simulink model "Hall_sensor_120deg_filter_org"  (R2024b)
settings: Solver=FixedStepAuto  StartTime=0.0  StopTime=1.5  FixedStep=1e-6  RelTol=1e-3
undefined symbols (not defined in the file): closed_loop, control_mode, D_duty_cycle, D_m, DiscIntNeverNeededParam, hall_errors, hall_errors_ON, I_duty_cycle, J_t, L_ss, lambda_m, P, P_duty_cycle, r_s, R_vs, T_m, theta_v, V_bus
libraries: spsMosfetLib x6, spsSeriesRLCBranchLib x4, spsVoltageMeasurementLib x3, spsControlledCurrentSourceLib x3, eeGeneralControl x2, slpidlib x2, embmathops x2, simulink x1, spsPWMGeneratorDCDCLib x1, spsDCVoltageSourceLib x1, sps_lib x1
settings Model: SimulationMode=accelerator  Creator=baolo  LastModifiedBy=baolo
settings SolverCC: ZeroCrossAlgorithm=Adaptive
settings DebuggingCC: IgnoredZcDiagnostic=none

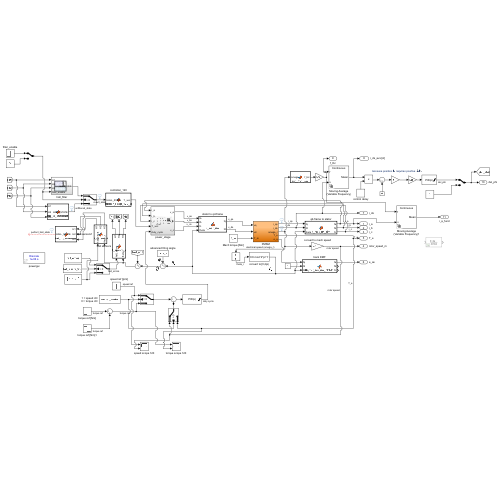
[thumbnail: Simulink's stored preview of the top-level diagram]
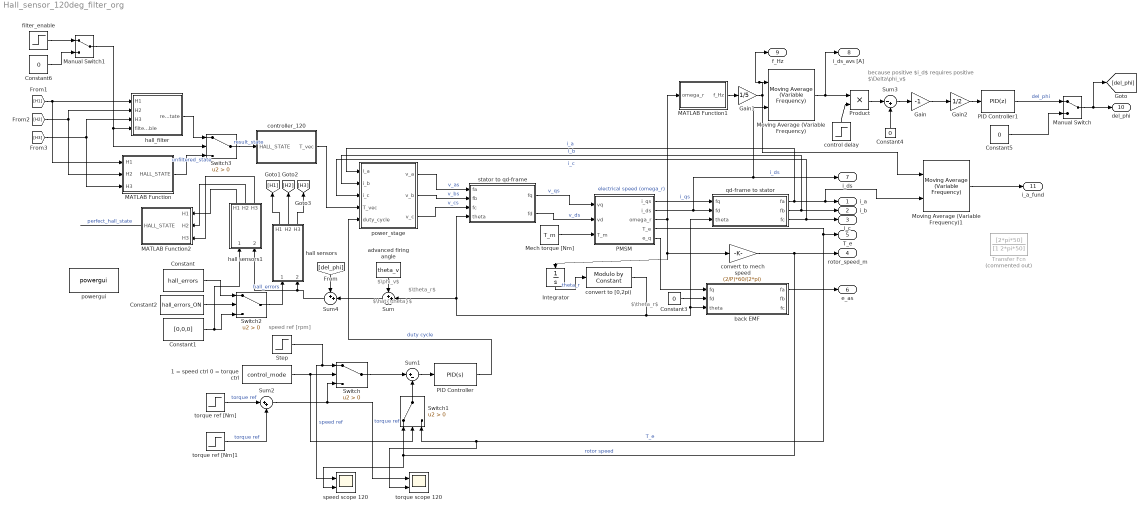
== system Hall_sensor_120deg_filter_org ==
  note: because positive $i_d$ requires positive $\Delta\phi_v$
  note: $\phi_v$
  note: speed ref [rpm]
  note: $\theta_r$
  note: $\theta_r$
  note: $\hat{\theta}$
  1 = speed ctrl 0 = torque ctrl : Constant  Value=control_mode
  Constant : Constant  Value=hall_errors
  Constant1 : Constant  Value=[0,0,0]
  Constant2 : Constant  Value=hall_errors_ON
  Constant{3..6} (4 alike) : Constant  Value=0
  Gain : Gain  Gain=-1
  Gain1 : Gain  Gain=1/5
  Gain2 : Gain  Gain=1/2
  Integrator : Integrator
  MATLAB Function : MATLAB Function  TreatAsAtomicUnit=on
  MATLAB Function1 : MATLAB Function  TreatAsAtomicUnit=on
  MATLAB Function2 : MATLAB Function  TreatAsAtomicUnit=on
  Manual Switch : ManualSwitch
  Manual Switch1 : ManualSwitch
  Mech torque [Nm] : Constant  Value=T_m
  Moving Average (Variable Frequency) : eeGeneralControl/Moving Average (Variable Frequency)  VariantControl=Variant1  LabelModeActiveChoice=Continuous  f0=60  fmin=0.1  x0=0  BufferSize=32768  Ts=0
      settings: LibrarySourceBlock=|
      | ee_sl_lib/General Control/Moving Average
      | (Variable Frequency)
  Moving Average (Variable Frequency)1 : eeGeneralControl/Moving Average (Variable Frequency)  VariantControl=Variant1  LabelModeActiveChoice=Continuous  f0=60  fmin=0.1  x0=0  BufferSize=32768  Ts=0
      settings: LibrarySourceBlock=|
      | ee_sl_lib/General Control/Moving Average
      | (Variable Frequency)
  PID Controller : slpidlib/PID Controller  Controller=PID  Form=Parallel  TimeDomain=Continuous-time  UseExternalTs=off  SampleTime=-1  IntegratorMethod=Forward Euler  FilterMethod=Forward Euler  ControllerParametersSource=internal  P=P_duty_cycle  I=I_duty_cycle  UseKiTs=off  D=D_duty_cycle  UseExternalDerivativeSource=off  N=100  UseFilter=on  TunerSelectOption=Transfer Function Based (PID Tuner App)  InitialConditionSource=internal  InitialConditionForIntegrator=0  InitialConditionForFilter=0  DifferentiatorICPrevScaledInput=0  ExternalReset=none  TrackingMode=off  Kt=1  LimitOutput=on  SatLimitsSource=internal  UpperSaturationLimit=1  LowerSaturationLimit=0  LinearizeAsGain=on  AntiWindupMode=none  Kb=1  LimitIntegrator=off  UpperIntegratorSaturationLimit=inf  LowerIntegratorSaturationLimit=-inf  POutMin=[]  POutMax=[]  IOutMin=[]  IOutMax=[]  DOutMin=[]  DOutMax=[]  NOutMin=[]  NOutMax=[]  SumOutMin=[]  SumOutMax=[]  SaturationOutMin=[]  SaturationOutMax=[]  PParamMin=[]  PParamMax=[]  IParamMin=[]  IParamMax=[]  DParamMin=[]  DParamMax=[]  NParamMin=[]  NParamMax=[]  KbParamMin=[]  KbParamMax=[]  KtParamMin=[]  KtParamMax=[]  KbOutMin=[]  KbOutMax=[]  KtOutMin=[]  KtOutMax=[]  IntegratorOutMin=[]  IntegratorOutMax=[]  FilterOutMin=[]  FilterOutMax=[]  SumI1OutMin=[]  SumI1OutMax=[]  SumI2OutMin=[]  SumI2OutMax=[]  SumI3OutMin=[]  SumI3OutMax=[]  SumI4OutMin=[]  SumI4OutMax=[]  SumDOutMin=[]  SumDOutMax=[]  DifferentiatorOutMin=[]  DifferentiatorOutMax=[]  FilterDiffOutCoefMin=[]  FilterDiffOutCoefMax=[]  ReciprocalOutMin=[]  ReciprocalOutMax=[]  SumDenOutMin=[]  SumDenOutMax=[]  SumNumOutMin=[]  SumNumOutMax=[]  DivideOutMin=[]  DivideOutMax=[]  UdiffTsProdOutMin=[]  UdiffTsProdOutMax=[]  NTsProdOutMin=[]  NTsProdOutMax=[]  UintegralTsProdOutMin=[]  UintegralTsProdOutMax=[]  UngainTsProdOutMin=[]  UngainTsProdOutMax=[]  ClampingZeroOutDataTypeStr=Inherit: Inherit via back propagation  ClampingZeroOutMin=[]  ClampingZeroOutMax=[]  FilterDenConstantOutDataTypeStr=Inherit: Inherit via back propagation  FilterDenConstantOutMin=[]  FilterDenConstantOutMax=[]  PCopyOutDataTypeStr=Inherit: Inherit via back propagation  PCopyOutMin=[]  PCopyOutMax=[]  NCopyOutDataTypeStr=Inherit: Inherit via back propagation  NCopyOutMin=[]  NCopyOutMax=[]  IntegratorContinuousStateAttributes=''  IntegratorStateMustResolveToSignalObject=off  IntegratorRTWStateStorageClass=Auto  FilterContinuousStateAttributes=''  FilterStateMustResolveToSignalObject=off  FilterRTWStateStorageClass=Auto  ParallelPVariant=InternalParameters  IdealPVariant=Disabled  IVariant=InternalParameters  DVariant=InternalParameters  IntegratorVariant=Continuous  SatVariant=Enabled  AWVariant=Passthrough  PCopyVariant=Disabled  TRVariant=Disabled  FdbkBlocksVariant=Forward  IdealPFdbkVariant=Disabled  SatFdbkVariant=Disabled  DerivativeFilterVariant=ContFilter  NVariant=InternalParameters  NCopyVariant=Disabled  FilterICVariant=InternalICsFilter  IntegratorICVariant=InternalICs  ExternalResetVariant=Disabled  TRSumVariant=Passthrough  SumFdbkVariant=Disabled  SumVariant=Sum_PID  TsampFilterVariant=InternalTs  TsampNgainVariant=Passthrough  TsampIntegralVariant=Disabled_SignalSpec  ExternalSaturationOutDataTypeStr=Inherit: Same as second input  DerivativeSourceVariant=ErrorSignal  PreIntVariant=InternalPreInt
  PID Controller1 : slpidlib/PID Controller  Controller=PID  Form=Parallel  TimeDomain=Discrete-time  UseExternalTs=off  SampleTime=-1  IntegratorMethod=Forward Euler  FilterMethod=Forward Euler  ControllerParametersSource=internal  P=0.0136  I=1.488  UseKiTs=off  D=0  UseExternalDerivativeSource=off  N=100  UseFilter=on  TunerSelectOption=Transfer Function Based (PID Tuner App)  InitialConditionSource=internal  InitialConditionForIntegrator=0  InitialConditionForFilter=0  DifferentiatorICPrevScaledInput=0  ExternalReset=none  TrackingMode=off  Kt=1  LimitOutput=on  SatLimitsSource=internal  UpperSaturationLimit=pi/3  LowerSaturationLimit=-pi/3  LinearizeAsGain=on  AntiWindupMode=none  Kb=1  LimitIntegrator=off  UpperIntegratorSaturationLimit=inf  LowerIntegratorSaturationLimit=-inf  POutMin=[]  POutMax=[]  IOutMin=[]  IOutMax=[]  DOutMin=[]  DOutMax=[]  NOutMin=[]  NOutMax=[]  SumOutMin=[]  SumOutMax=[]  SaturationOutMin=[]  SaturationOutMax=[]  PParamMin=[]  PParamMax=[]  IParamMin=[]  IParamMax=[]  DParamMin=[]  DParamMax=[]  NParamMin=[]  NParamMax=[]  KbParamMin=[]  KbParamMax=[]  KtParamMin=[]  KtParamMax=[]  KbOutMin=[]  KbOutMax=[]  KtOutMin=[]  KtOutMax=[]  IntegratorOutMin=[]  IntegratorOutMax=[]  FilterOutMin=[]  FilterOutMax=[]  SumI1OutMin=[]  SumI1OutMax=[]  SumI2OutMin=[]  SumI2OutMax=[]  SumI3OutMin=[]  SumI3OutMax=[]  SumI4OutMin=[]  SumI4OutMax=[]  SumDOutMin=[]  SumDOutMax=[]  DifferentiatorOutMin=[]  DifferentiatorOutMax=[]  FilterDiffOutCoefMin=[]  FilterDiffOutCoefMax=[]  ReciprocalOutMin=[]  ReciprocalOutMax=[]  SumDenOutMin=[]  SumDenOutMax=[]  SumNumOutMin=[]  SumNumOutMax=[]  DivideOutMin=[]  DivideOutMax=[]  UdiffTsProdOutMin=[]  UdiffTsProdOutMax=[]  NTsProdOutMin=[]  NTsProdOutMax=[]  UintegralTsProdOutMin=[]  UintegralTsProdOutMax=[]  UngainTsProdOutMin=[]  UngainTsProdOutMax=[]  ClampingZeroOutDataTypeStr=Inherit: Inherit via back propagation  ClampingZeroOutMin=[]  ClampingZeroOutMax=[]  FilterDenConstantOutDataTypeStr=Inherit: Inherit via back propagation  FilterDenConstantOutMin=[]  FilterDenConstantOutMax=[]  PCopyOutDataTypeStr=Inherit: Inherit via back propagation  PCopyOutMin=[]  PCopyOutMax=[]  NCopyOutDataTypeStr=Inherit: Inherit via back propagation  NCopyOutMin=[]  NCopyOutMax=[]  IntegratorContinuousStateAttributes=''  IntegratorStateMustResolveToSignalObject=off  IntegratorRTWStateStorageClass=Auto  FilterContinuousStateAttributes=''  FilterStateMustResolveToSignalObject=off  FilterRTWStateStorageClass=Auto  ParallelPVariant=InternalParameters  IdealPVariant=Disabled  IVariant=InternalParameters  DVariant=InternalParameters  IntegratorVariant=Discrete  SatVariant=Enabled  AWVariant=Passthrough  PCopyVariant=Disabled  TRVariant=Disabled  FdbkBlocksVariant=Forward  IdealPFdbkVariant=Disabled  SatFdbkVariant=Disabled  DerivativeFilterVariant=ForwardEulerFilter  NVariant=InternalParameters  NCopyVariant=Disabled  FilterICVariant=InternalICsFilter  IntegratorICVariant=InternalICs  ExternalResetVariant=Disabled  TRSumVariant=Passthrough  SumFdbkVariant=Disabled  SumVariant=Sum_PID  TsampFilterVariant=InternalTs  TsampNgainVariant=Passthrough  TsampIntegralVariant=Disabled_SignalSpec  ExternalSaturationOutDataTypeStr=Inherit: Same as second input  DerivativeSourceVariant=ErrorSignal  PreIntVariant=InternalPreInt
  PMSM : Subsystem
  Product : Product
  Step : Step  Time=0.1  After=1000  SampleTime=0
  Sum : Sum  Inputs=++|
  Sum1 : Sum  Inputs=|+-
  Sum2 : Sum  Inputs=|++
  Sum3 : Sum  Inputs=|-+
  Sum4 : Sum  Inputs=++|
  Switch{,1..3} (4 alike) : Switch  Criteria=u2 > Threshold  SaturateOnIntegerOverflow=off  InputSameDT=off
  Transfer Fcn : TransferFcn  Commented=on  Numerator=[2*pi*50]  Denominator=[1 2*pi*50]
  advanced firing angle : Constant  Value=theta_v
  back EMF : MATLAB Function  TreatAsAtomicUnit=on
  control delay : Step  Time=0.7  SampleTime=0
  controller_120 : MATLAB Function  TreatAsAtomicUnit=on
  convert to [0,2pi) : embmathops/Modulo by Constant  Denominator=2*pi  SimulateUsing=Code generation
      settings: LibrarySourceBlock=embeddedMathLib/Modulo by Constant
  convert to mech speed : Gain  Gain=(2/P)*60/(2*pi)
  filter_enable : Step  Time=0.5  SampleTime=0
  hall sensors : MATLAB Function  TreatAsAtomicUnit=on
  hall sensors1 : MATLAB Function  TreatAsAtomicUnit=on
  hall_filter : Subsystem
  power_stage : Subsystem
  powergui : sps_lib/powergui  Priority=1  SimulationMode=Discrete  SampleTime=1e-6  frequency=60  Iterations=50  frequencyindice=0  Pbase=100e6  ErrMax=1e-4  UnitsV=kV  UnitsW=MW  buscounter=0  FunctionMessages=off  echomessages=off  EnableUseOfTLC=off  CurrentSourceSwitches=off  DisableSnubberDevices=off  DisableRonSwitches=off  DisableVfSwitches=off  DisplayEquations=off  AutomaticDiscreteSolvers=off  SolverType=Tustin/Backward Euler (TBE)  Interpol=off  ExternalGateDelay=off  methode=off  Ts=100  x0status=blocks  SPID=on  SwTol=0  HookPort=off  NonlinearTolerance=1e-4  nMaxIteration=100  ContinueOnMaxIteration=off  RestoreLinks=warning  ResistiveCurrentMeasurement=off  Frange=[0:2:500]  Ylog=off  Xlog=on  ShowGrid=off  save=off  variable=ZData  structure=0  ZoomFFT=off  StartTime=0.0  cycles=1  DisplayStyle=1  fundamental=60  FreqAxis=off  MaxFrequency=1000  frequencyindicesteady=1  RmsSteady=1  display=off
  qd-frame to stator : MATLAB Function  TreatAsAtomicUnit=on
  speed scope 120 : Scope  NumInputPorts=2
  stator to qd-frame : MATLAB Function  TreatAsAtomicUnit=on
  torque ref [Nm] : Step  Time=0.1  After=1e-1  SampleTime=0  ZeroCross=off
  torque ref [Nm]1 : Step  After=-0.5e-1  SampleTime=0
  torque scope 120 : Scope  NumInputPorts=2
  i_a : Outport
  i_b : Outport  Port=2
  i_c : Outport  Port=3
  rotor_speed_m : Outport  Port=4
  T_e : Outport  Port=5
  e_as : Outport  Port=6
  i_ds : Outport  Port=7
  i_ds_avs [A] : Outport  Port=8
  f_Hz : Outport  Port=9
  del_phi : Outport  Port=10
  i_a_fund : Outport  Port=11
  wires:
  stator to qd-frame/1(fq) -> PMSM/1(vq)  "v_qs"
  stator to qd-frame/2(fd) -> PMSM/2(vd)  "v_ds"
  Mech torque [Nm]/1 -> PMSM/3(T_m)
  PMSM/1(i_qs) -> qd-frame to stator/1(fq)  "i_qs"
  PMSM/2(i_ds) -> i_ds/1, Moving Average (Variable Frequency)/2, qd-frame to stator/2(fd)  "i_ds"
  PMSM/3(omega_r) -> MATLAB Function1/1(omega_r), convert to mech speed/1, Integrator/1  "electrical speed (omega_r)"
  convert to [0,2pi)/1 -> stator to qd-frame/4(theta), Sum/2, back EMF/3(theta), qd-frame to stator/3(theta)
  power_stage/1(v_a) -> stator to qd-frame/1(fa)  "v_as"
  power_stage/2(v_b) -> stator to qd-frame/2(fb)  "v_bs"
  power_stage/3(v_c) -> stator to qd-frame/3(fc)  "v_cs"
  Integrator/1 -> convert to [0,2pi)/1  "theta_r"
  hall sensors/1(H1) -> [H1]
  hall sensors/2(H2) -> [H2]
  hall sensors/3(H3) -> [H3]
  advanced firing angle/1 -> Sum/1
  Sum/1 -> Sum4/2
  qd-frame to stator/1(fa) -> power_stage/1(i_a), Moving Average (Variable Frequency)1/2, i_a/1  "i_a"
  qd-frame to stator/2(fb) -> power_stage/2(i_b), i_b/1  "i_b"
  qd-frame to stator/3(fc) -> power_stage/3(i_c), i_c/1  "i_c"
  convert to mech speed/1 -> rotor_speed_m/1, speed scope 120/2, Switch1/1  "rotor speed"
  PMSM/4(T_e) -> torque scope 120/2, Switch1/3, T_e/1  "T_e"
  1 = speed ctrl 0 = torque ctrl/1 -> Switch/2, Switch1/2
  Step/1 -> speed scope 120/1, Switch/1  "speed ref"
  Sum2/1 -> torque scope 120/1, Switch/3  "torque ref"
  Switch1/1 -> Sum1/2
  Switch/1 -> Sum1/1
  Sum1/1 -> PID Controller/1
  PID Controller/1 -> power_stage/5(duty_cycle)  "duty cycle"
  torque ref [Nm]/1 -> Sum2/1  "torque ref"
  torque ref [Nm]1/1 -> Sum2/2  "torque ref"
  Constant/1 -> Switch2/1
  Switch2/1 -> hall sensors/1(hall_errors)  "hall_errors"
  Constant1/1 -> hall sensors1/1(hall_errors), Switch2/3
  controller_120/1(T_vec) -> power_stage/4(T_vec)
  Constant2/1 -> Switch2/2
  PMSM/5(e_q) -> back EMF/1(fq)
  Constant3/1 -> back EMF/2(fd)
  back EMF/1(fa) -> e_as/1
  Moving Average (Variable Frequency)/1 -> Product/1, i_ds_avs [A]/1
  Gain1/1 -> Moving Average (Variable Frequency)1/1, f_Hz/1, Moving Average (Variable Frequency)/1
  Constant4/1 -> Sum3/2
  Sum3/1 -> Gain/1
  PID Controller1/1 -> Manual Switch/1  "del_phi"
  [del_phi] -> Sum4/1
  Sum4/1 -> hall sensors1/2(theta_r), hall sensors/2(theta_r)
  Constant5/1 -> Manual Switch/2
  control delay/1 -> Product/2
  Product/1 -> Sum3/1
  Manual Switch/1 -> del_phi/1, [del_phi]
  Gain/1 -> Gain2/1
  [H1] -> hall_filter/1(H1), MATLAB Function/1(H1)
  [H2] -> hall_filter/2(H2), MATLAB Function/2(H2)
  [H3] -> hall_filter/3(H3), MATLAB Function/3(H3)
  MATLAB Function/1(HALL_STATE) -> Switch3/3  "unfiltered_state"
  Switch3/1 -> controller_120/1(HALL_STATE)  "result_state"
  Manual Switch1/1 -> Switch3/2, hall_filter/4(filter_enable)
  filter_enable/1 -> Manual Switch1/1
  Constant6/1 -> Manual Switch1/2
  hall sensors1/1(H1) -> MATLAB Function2/1(H1)
  hall sensors1/2(H2) -> MATLAB Function2/2(H2)
  hall sensors1/3(H3) -> MATLAB Function2/3(H3)
  MATLAB Function2/1(HALL_STATE) -> ?  "perfect_hall_state"
  hall_filter/1(result_state) -> Switch3/1
  MATLAB Function1/1(f_Hz) -> Gain1/1
  Gain2/1 -> PID Controller1/1
  Moving Average (Variable Frequency)1/1 -> i_a_fund/1

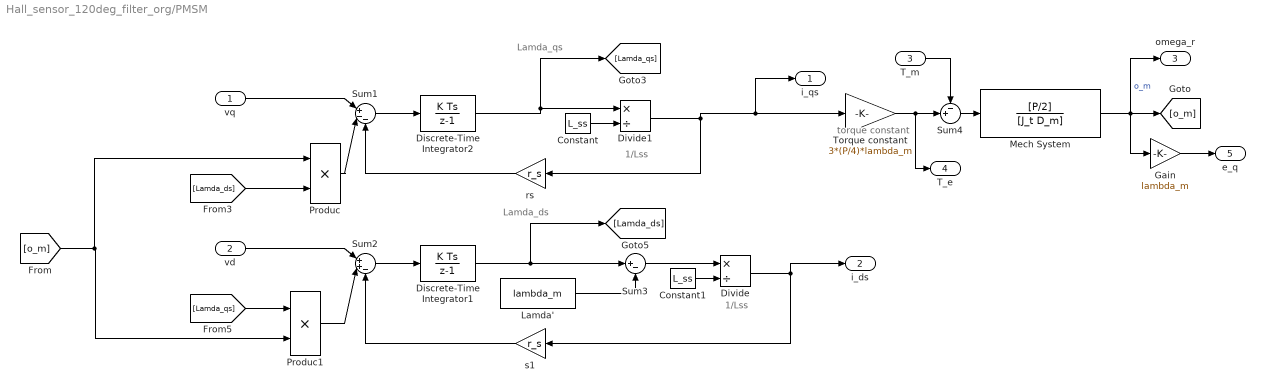
== system Hall_sensor_120deg_filter_org/PMSM ==
  note: torque constant
  note: Lamda_ds
  note: Lamda_qs
  note: 1/Lss
  note: 1/Lss
  vq : Inport
  vd : Inport  Port=2
  T_m : Inport  Port=3
  Constant : Constant  Value=L_ss
  Constant1 : Constant  Value=L_ss
  Discrete-Time Integrator1 : DiscreteIntegrator  SampleTime=-1  ICPrevOutput=DiscIntNeverNeededParam  ICPrevScaledInput=DiscIntNeverNeededParam
  Discrete-Time Integrator2 : DiscreteIntegrator  SampleTime=-1  ICPrevOutput=DiscIntNeverNeededParam  ICPrevScaledInput=DiscIntNeverNeededParam
  Divide : Product  Inputs=*/
  Divide1 : Product  Inputs=*/
  Gain : Gain  Gain=lambda_m
  Lamda' : Constant  Value=lambda_m
  Mech System : TransferFcn  Numerator=[P/2]  Denominator=[J_t D_m]
  Produc : Product  RndMeth=Zero
  Produc1 : Product  RndMeth=Zero
  Sum1 : Sum  Inputs=|+--
  Sum2 : Sum  Inputs=|++-
  Sum3 : Sum  Inputs=|+-
  Sum4 : Sum  Inputs=-+|
  Torque constant : Gain  Gain=3*(P/4)*lambda_m
  rs : Gain  Gain=r_s
  s1 : Gain  Gain=r_s
  i_qs : Outport
  i_ds : Outport  Port=2
  omega_r : Outport  Port=3
  T_e : Outport  Port=4
  e_q : Outport  Port=5
  wires:
  vd/1 -> Sum2/1
  vq/1 -> Sum1/1
  [Lamda_qs] -> Produc1/1
  [Lamda_ds] -> Produc/2
  [o_m] -> Produc1/2, Produc/1
  Lamda'/1 -> Sum3/2
  Sum3/1 -> Divide/1
  s1/1 -> Sum2/3
  Discrete-Time Integrator1/1 -> [Lamda_ds], Sum3/1
  Sum2/1 -> Discrete-Time Integrator1/1
  Produc1/1 -> Sum2/2
  Divide1/1 -> i_qs/1, Torque constant/1, rs/1
  rs/1 -> Sum1/3
  Discrete-Time Integrator2/1 -> [Lamda_qs], Divide1/1
  Sum1/1 -> Discrete-Time Integrator2/1
  Produc/1 -> Sum1/2
  Torque constant/1 -> Sum4/2, T_e/1
  Divide/1 -> i_ds/1, s1/1
  T_m/1 -> Sum4/1
  Sum4/1 -> Mech System/1
  Constant/1 -> Divide1/2
  Constant1/1 -> Divide/2
  Mech System/1 -> Gain/1, omega_r/1, [o_m]  "o_m"
  Gain/1 -> e_q/1

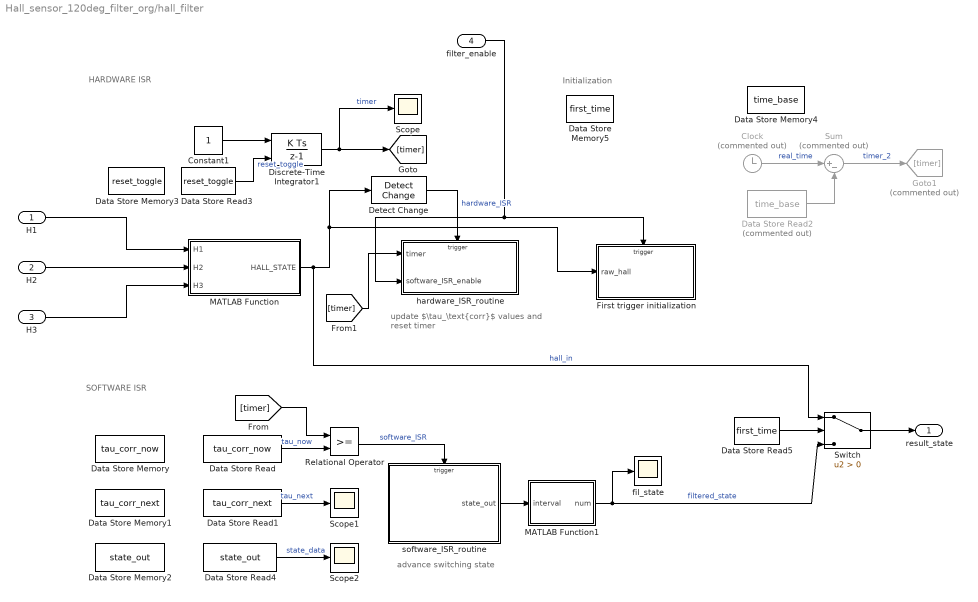
== system Hall_sensor_120deg_filter_org/hall_filter ==
  note: Initialization
  note: SOFTWARE ISR
  note: HARDWARE ISR
  note: update $\tau_\text{corr}$ values and reset timer
  note: advance switching state
  H1 : Inport
  H2 : Inport  Port=2
  H3 : Inport  Port=3
  filter_enable : Inport  Port=4
  Clock : Clock  Commented=on
  Constant1 : Constant
  Data Store Memory : DataStoreMemory  DataStoreName=tau_corr_now  WriteAfterWriteMsg=warning  InitialValue=-1  ShowAdditionalParam=off
  Data Store Memory1 : DataStoreMemory  DataStoreName=tau_corr_next  WriteAfterWriteMsg=warning  InitialValue=-1  ShowAdditionalParam=off
  Data Store Memory2 : DataStoreMemory  DataStoreName=state_out  WriteAfterWriteMsg=warning  InitialValue=2  ShowAdditionalParam=off
  Data Store Memory3 : DataStoreMemory  DataStoreName=reset_toggle  WriteAfterWriteMsg=warning  ShowAdditionalParam=off
  Data Store Memory4 : DataStoreMemory  DataStoreName=time_base  WriteAfterWriteMsg=warning  ShowAdditionalParam=off
  Data Store Memory5 : DataStoreMemory  DataStoreName=first_time  WriteAfterWriteMsg=warning  InitialValue=1  ShowAdditionalParam=off
  Data Store Read : DataStoreRead  DataStoreName=tau_corr_now  IndexOptions=Index vector (dialog)  Indices=1  OutputSizes=1
  Data Store Read1 : DataStoreRead  DataStoreName=tau_corr_next  IndexOptions=Index vector (dialog)  Indices=1  OutputSizes=1
  Data Store Read2 : DataStoreRead  Commented=on  DataStoreName=time_base  IndexOptions=Index vector (dialog)  Indices=1  OutputSizes=1
  Data Store Read3 : DataStoreRead  DataStoreName=reset_toggle  IndexOptions=Index vector (dialog)  Indices=1  OutputSizes=1
  Data Store Read4 : DataStoreRead  DataStoreName=state_out  IndexOptions=Index vector (dialog)  Indices=1  OutputSizes=1
  Data Store Read5 : DataStoreRead  DataStoreName=first_time  IndexOptions=Index vector (dialog)  Indices=1  OutputSizes=1
  Detect Change : simulink/Logic and Bit Operations/Detect Change  vinit=0  OutDataTypeStr=boolean
  Discrete-Time Integrator1 : DiscreteIntegrator  ExternalReset=either  SampleTime=1/(1e6)  ICPrevOutput=DiscIntNeverNeededParam  ICPrevScaledInput=DiscIntNeverNeededParam
  First trigger initialization : Subsystem  TreatAsAtomicUnit=on
  Goto1 : Goto  Commented=on  GotoTag=timer
  MATLAB Function : MATLAB Function  TreatAsAtomicUnit=on
  MATLAB Function1 : MATLAB Function  TreatAsAtomicUnit=on
  Relational Operator : RelationalOperator  OutDataTypeStr=boolean  RndMeth=Simplest  InputSameDT=off
  Scope : Scope
  Scope1 : Scope
  Scope2 : Scope
  Sum : Sum  Commented=on  Inputs=|+-
  Switch : Switch  Criteria=u2 > Threshold  SaturateOnIntegerOverflow=off  InputSameDT=off
  fil_state : Scope
  hardware_ISR_routine : Subsystem  Priority=1
  software_ISR_routine : Subsystem  Priority=10  TreatAsAtomicUnit=on
  result_state : Outport
  wires:
  Discrete-Time Integrator1/1 -> [timer], Scope/1  "timer"
  Relational Operator/1 -> software_ISR_routine/Trigger  "software_ISR"
  Constant1/1 -> Discrete-Time Integrator1/1
  [timer] -> Relational Operator/1
  software_ISR_routine/1(state_out) -> MATLAB Function1/1(interval)
  MATLAB Function/1(HALL_STATE) -> Switch/1, Detect Change/1, First trigger initialization/1(raw_hall)  "hall_in"
  Data Store Read3/1 -> Discrete-Time Integrator1/2  "reset_toggle"
  Data Store Read1/1 -> Scope1/1  "tau_next"
  Data Store Read/1 -> Relational Operator/2  "tau_now"
  H3/1 -> MATLAB Function/3(H3)
  H2/1 -> MATLAB Function/2(H2)
  H1/1 -> MATLAB Function/1(H1)
  MATLAB Function1/1(num) -> fil_state/1, Switch/3  "filtered_state"
  Detect Change/1 -> hardware_ISR_routine/Trigger  "hardware_ISR"
  Data Store Read4/1 -> Scope2/1  "state_data"
  filter_enable/1 -> First trigger initialization/Trigger, hardware_ISR_routine/2(software_ISR_enable)
  Clock/1 -> Sum/1  "real_time"
  [timer] -> hardware_ISR_routine/1(timer)
  Data Store Read2/1 -> Sum/2
  Sum/1 -> Goto1/1  "timer_2"
  Data Store Read5/1 -> Switch/2
  Switch/1 -> result_state/1

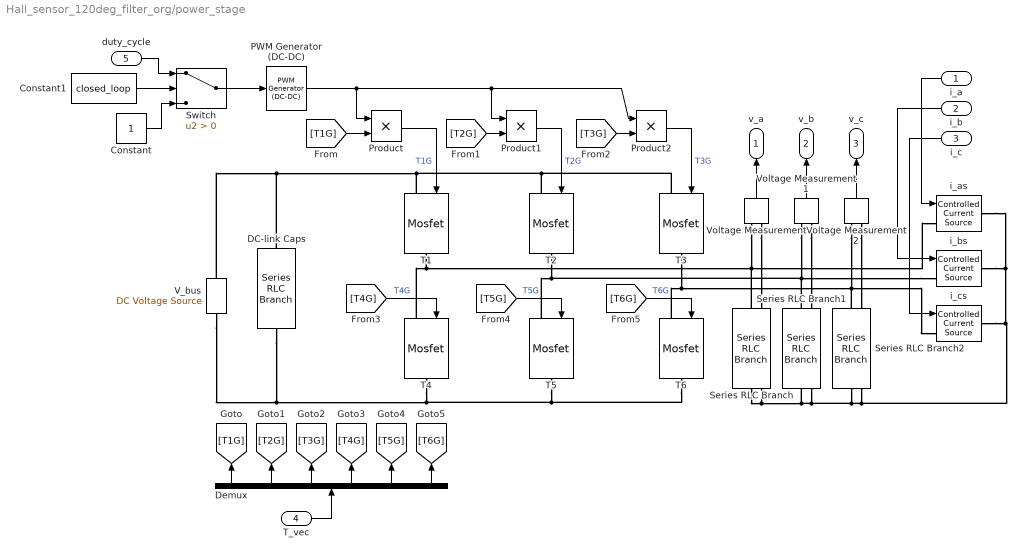
== system Hall_sensor_120deg_filter_org/power_stage ==
  i_a : Inport
  i_b : Inport  Port=2
  i_c : Inport  Port=3
  T_vec : Inport  Port=4
  duty_cycle : Inport  Port=5
  Constant : Constant
  Constant1 : Constant  Value=closed_loop
  DC-link Caps : spsSeriesRLCBranchLib/Series RLC Branch  LConnTagsString=__new0  RConnTagsString=__new0  BranchType=RC  Resistance=1e-6  Inductance=0  SetiL0=off  InitialCurrent=0  Capacitance=100e-6  Setx0=off  InitialVoltage=0  Measurements=None
  Demux : Demux  Outputs=6
  PWM Generator (DC-DC) : spsPWMGeneratorDCDCLib/PWM Generator (DC-DC)  Fsw=f_SW_Hz  Ts=0
  Product : Product
  Product1 : Product
  Product2 : Product
  Series RLC Branch : spsSeriesRLCBranchLib/Series RLC Branch  LConnTagsString=__new0  RConnTagsString=__new0  BranchType=R  Resistance=R_vs  Inductance=0  SetiL0=off  InitialCurrent=0  Capacitance=inf  Setx0=off  InitialVoltage=0  Measurements=None
  Series RLC Branch1 : spsSeriesRLCBranchLib/Series RLC Branch  LConnTagsString=__new0  RConnTagsString=__new0  BranchType=R  Resistance=R_vs  Inductance=0  SetiL0=off  InitialCurrent=0  Capacitance=inf  Setx0=off  InitialVoltage=0  Measurements=None
  Series RLC Branch2 : spsSeriesRLCBranchLib/Series RLC Branch  LConnTagsString=__new0  RConnTagsString=__new0  BranchType=R  Resistance=R_vs  Inductance=0  SetiL0=off  InitialCurrent=0  Capacitance=inf  Setx0=off  InitialVoltage=0  Measurements=None
  Switch : Switch  Criteria=u2 > Threshold  SaturateOnIntegerOverflow=off  InputSameDT=off
  T{1..6} (6 alike) : spsMosfetLib/Mosfet  Ron=R_dsON_Ohm  Lon=0  Rd=0.01  Vfd=0.7  IC=0  Rs=1e5  Cs=inf  Measurements=off
  V_bus : spsDCVoltageSourceLib/DC Voltage Source  Amplitude=V_bus  Measurements=None
  Voltage Measurement : spsVoltageMeasurementLib/Voltage Measurement  PhasorSimulation=off  OutputType=Complex  PSBequivalent=0
  Voltage Measurement1 : spsVoltageMeasurementLib/Voltage Measurement  PhasorSimulation=off  OutputType=Complex  PSBequivalent=0
  Voltage Measurement2 : spsVoltageMeasurementLib/Voltage Measurement  PhasorSimulation=off  OutputType=Complex  PSBequivalent=0
  i_as : spsControlledCurrentSourceLib/Controlled Current Source  Initialize=on  Source_Type=AC  Amplitude=0  Phase=0  Frequency=0  Measurements=None
  i_bs : spsControlledCurrentSourceLib/Controlled Current Source  Initialize=on  Source_Type=AC  Amplitude=0  Phase=0  Frequency=0  Measurements=None
  i_cs : spsControlledCurrentSourceLib/Controlled Current Source  Initialize=on  Source_Type=AC  Amplitude=0  Phase=0  Frequency=0  Measurements=None
  v_a : Outport
  v_b : Outport  Port=2
  v_c : Outport  Port=3
  wires:
  T_vec/1 -> Demux/1
  Product1/1 -> T2/1  "T2G"
  PWM Generator (DC-DC)/1 -> Product/1, Product2/1, Product1/1
  Demux/6 -> [T6G]
  [T4G] -> T4/1  "T4G"
  [T5G] -> T5/1  "T5G"
  Demux/4 -> [T4G]
  Voltage Measurement/1 -> v_a/1
  [T2G] -> Product1/2
  Voltage Measurement1/1 -> v_b/1
  Voltage Measurement2/1 -> v_c/1
  i_a/1 -> i_as/1
  Demux/1 -> [T1G]
  Demux/5 -> [T5G]
  [T6G] -> T6/1  "T6G"
  i_c/1 -> i_cs/1
  Product/1 -> T1/1  "T1G"
  [T3G] -> Product2/2
  i_b/1 -> i_bs/1
  Product2/1 -> T3/1  "T3G"
  Demux/2 -> [T2G]
  Demux/3 -> [T3G]
  [T1G] -> Product/2
  duty_cycle/1 -> Switch/1
  Constant/1 -> Switch/3
  Constant1/1 -> Switch/2
  Switch/1 -> PWM Generator (DC-DC)/1
  connections:
  i_bs/LConn1 -- Voltage Measurement1/LConn1 -- Series RLC Branch1/LConn1 -- T2/RConn1 -- T5/LConn1
  DC-link Caps/RConn1 -- V_bus/LConn1 -- T4/RConn1 -- T6/RConn1 -- T5/RConn1
  DC-link Caps/LConn1 -- V_bus/RConn1 -- T1/LConn1 -- T3/LConn1 -- T2/LConn1
  T4/LConn1 -- T1/RConn1 -- Voltage Measurement/LConn1 -- Series RLC Branch/LConn1 -- i_as/LConn1
  T3/RConn1 -- T6/LConn1 -- Voltage Measurement2/LConn1 -- Series RLC Branch2/LConn1 -- i_cs/LConn1
  Series RLC Branch/RConn1 -- Voltage Measurement/LConn2 -- i_bs/RConn1 -- i_as/RConn1 -- i_cs/RConn1 -- Voltage Measurement2/LConn2 -- Series RLC Branch2/RConn1 -- Voltage Measurement1/LConn2 -- Series RLC Branch1/RConn1

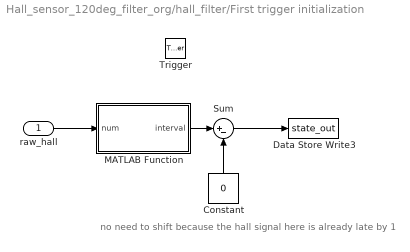
== system Hall_sensor_120deg_filter_org/hall_filter/First trigger initialization ==
  note: no need to shift because the hall signal here is already late by 1
  raw_hall : Inport
  Trigger : TriggerPort  VariantControl=(inherit)  PortDimensions=1
  Constant : Constant  Value=0
  Data Store Write3 : DataStoreWrite  DataStoreName=state_out  IndexOptions=Index vector (dialog)  Indices=1  OutputSizes=1
  MATLAB Function : MATLAB Function  TreatAsAtomicUnit=on
  Sum : Sum  Inputs=|+-
  wires:
  raw_hall/1 -> MATLAB Function/1(num)
  MATLAB Function/1(interval) -> Sum/1
  Sum/1 -> Data Store Write3/1
  Constant/1 -> Sum/2

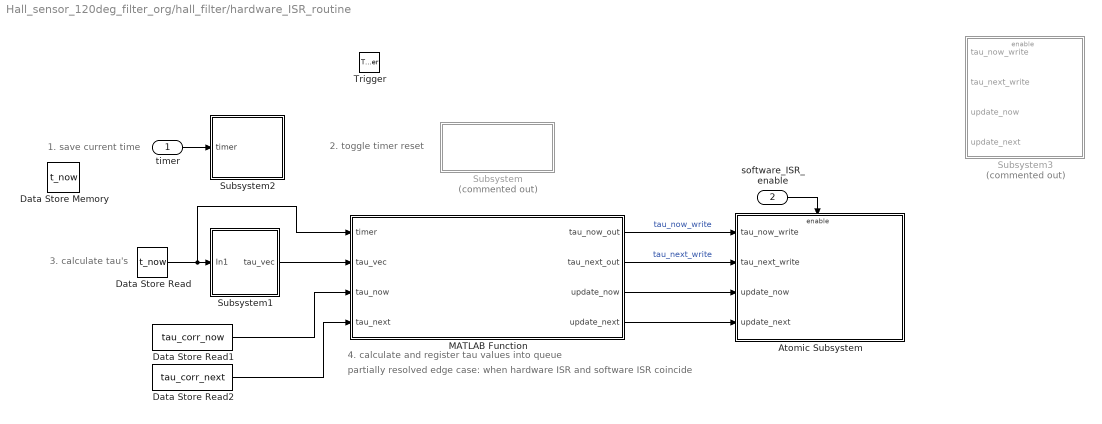
== system Hall_sensor_120deg_filter_org/hall_filter/hardware_ISR_routine ==
  note: partially resolved edge case: when hardware ISR and software ISR coincide
  note: 2. toggle timer reset
  note: 3. calculate tau's
  note: 4. calculate and register tau values into queue
  note: 1. save current time
  timer : Inport
  software_ISR_enable : Inport  Port=2
  Trigger : TriggerPort  VariantControl=(inherit)  PortDimensions=1
  Atomic Subsystem : Subsystem  Priority=5  TreatAsAtomicUnit=on
  Data Store Memory : DataStoreMemory  DataStoreName=t_now  WriteAfterWriteMsg=warning  ShowAdditionalParam=off
  Data Store Read : DataStoreRead  DataStoreName=t_now  IndexOptions=Index vector (dialog)  Indices=1  OutputSizes=1
  Data Store Read1 : DataStoreRead  DataStoreName=tau_corr_now  IndexOptions=Index vector (dialog)  Indices=1  OutputSizes=1
  Data Store Read2 : DataStoreRead  DataStoreName=tau_corr_next  IndexOptions=Index vector (dialog)  Indices=1  OutputSizes=1
  MATLAB Function : MATLAB Function  Priority=4  TreatAsAtomicUnit=on
  Subsystem : Subsystem  Priority=2  Commented=on
  Subsystem1 : Subsystem  Priority=3
  Subsystem2 : Subsystem  Priority=1
  Subsystem3 : Subsystem  Priority=5  Commented=on
  wires:
  Data Store Read/1 -> MATLAB Function/1(timer), Subsystem1/1(In1)
  Data Store Read1/1 -> MATLAB Function/3(tau_now)
  Data Store Read2/1 -> MATLAB Function/4(tau_next)
  timer/1 -> Subsystem2/1(timer)
  Subsystem1/1(tau_vec) -> MATLAB Function/2(tau_vec)
  MATLAB Function/1(tau_now_out) -> Atomic Subsystem/1(tau_now_write)  "tau_now_write"
  MATLAB Function/2(tau_next_out) -> Atomic Subsystem/2(tau_next_write)  "tau_next_write"
  software_ISR_enable/1 -> Atomic Subsystem/Enable
  MATLAB Function/3(update_now) -> Atomic Subsystem/3(update_now)
  MATLAB Function/4(update_next) -> Atomic Subsystem/4(update_next)

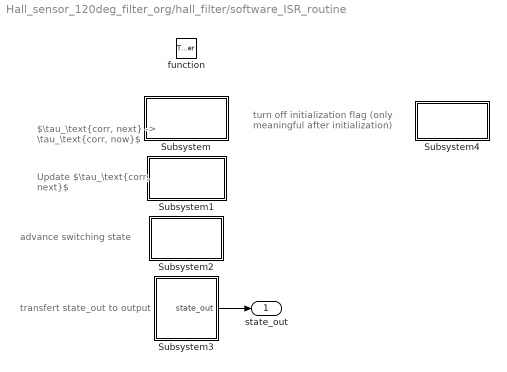
== system Hall_sensor_120deg_filter_org/hall_filter/software_ISR_routine ==
  note: turn off initialization flag
      | (only meaningful after initialization)
  note: advance switching state
  note: $\tau_\text{corr, next} -> \tau_\text{corr, now}$
  note: Update $\tau_\text{corr, next}$
  note: transfert state_out to output
  function : TriggerPort  VariantControl=(inherit)
  Subsystem : Subsystem  Priority=11
  Subsystem1 : Subsystem  Priority=12
  Subsystem2 : Subsystem  Priority=13
  Subsystem3 : Subsystem  Priority=14
  Subsystem4 : Subsystem  Priority=11
  state_out : Outport
  wires:
  Subsystem3/1(state_out) -> state_out/1

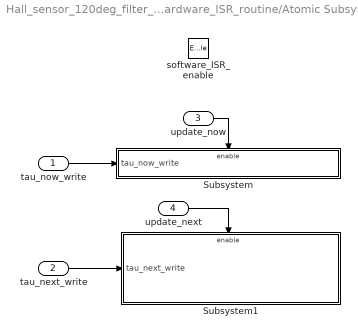
== system Hall_sensor_120deg_filter_org/hall_filter/hardware_ISR_routine/Atomic Subsystem ==
  tau_now_write : Inport
  tau_next_write : Inport  Port=2
  update_now : Inport  Port=3
  update_next : Inport  Port=4
  software_ISR_enable : EnablePort
  Subsystem : Subsystem
  Subsystem1 : Subsystem
  wires:
  tau_next_write/1 -> Subsystem1/1(tau_next_write)
  update_now/1 -> Subsystem/Enable
  update_next/1 -> Subsystem1/Enable
  tau_now_write/1 -> Subsystem/1(tau_now_write)

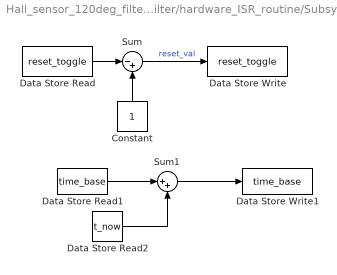
== system Hall_sensor_120deg_filter_org/hall_filter/hardware_ISR_routine/Subsystem ==
  Constant : Constant
  Data Store Read : DataStoreRead  DataStoreName=reset_toggle  IndexOptions=Index vector (dialog)  Indices=1  OutputSizes=1
  Data Store Read1 : DataStoreRead  DataStoreName=time_base  IndexOptions=Index vector (dialog)  Indices=1  OutputSizes=1
  Data Store Read2 : DataStoreRead  DataStoreName=t_now  IndexOptions=Index vector (dialog)  Indices=1  OutputSizes=1
  Data Store Write : DataStoreWrite  DataStoreName=reset_toggle  IndexOptions=Index vector (dialog)  Indices=1  OutputSizes=1
  Data Store Write1 : DataStoreWrite  DataStoreName=time_base  IndexOptions=Index vector (dialog)  Indices=1  OutputSizes=1
  Sum : Sum  Inputs=|-+
  Sum1 : Sum  Inputs=|++
  wires:
  Sum/1 -> Data Store Write/1  "reset_val"
  Data Store Read/1 -> Sum/1
  Constant/1 -> Sum/2
  Data Store Read1/1 -> Sum1/1
  Sum1/1 -> Data Store Write1/1
  Data Store Read2/1 -> Sum1/2

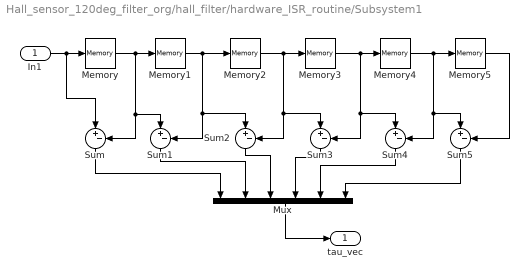
== system Hall_sensor_120deg_filter_org/hall_filter/hardware_ISR_routine/Subsystem1 ==
  In1 : Inport
  Memory{,1..5} (6 alike) : Memory  InheritSampleTime=on
  Mux : Mux  Inputs=6
  Sum{,1..5} (6 alike) : Sum  Inputs=|+-
  tau_vec : Outport
  wires:
  Memory1/1 -> Sum1/2, Sum2/1, Memory2/1
  Memory/1 -> Sum1/1, Sum/2, Memory1/1
  Memory2/1 -> Sum3/1, Sum2/2, Memory3/1
  In1/1 -> Sum/1, Memory/1
  Memory3/1 -> Sum4/1, Sum3/2, Memory4/1
  Memory4/1 -> Memory5/1, Sum5/1, Sum4/2
  Mux/1 -> tau_vec/1
  Memory5/1 -> Sum5/2
  Sum/1 -> Mux/1
  Sum1/1 -> Mux/2
  Sum2/1 -> Mux/3
  Sum3/1 -> Mux/4
  Sum4/1 -> Mux/5
  Sum5/1 -> Mux/6

== system Hall_sensor_120deg_filter_org/hall_filter/hardware_ISR_routine/Subsystem2 ==
  timer : Inport
  Data Store Write2 : DataStoreWrite  DataStoreName=t_now  IndexOptions=Index vector (dialog)  Indices=1  OutputSizes=1
  wires:
  timer/1 -> Data Store Write2/1

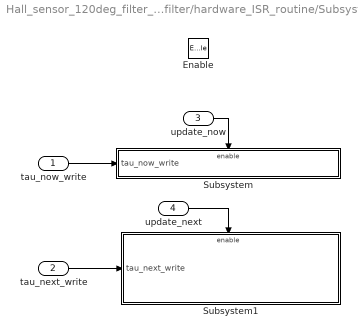
== system Hall_sensor_120deg_filter_org/hall_filter/hardware_ISR_routine/Subsystem3 ==
  tau_now_write : Inport
  tau_next_write : Inport  Port=2
  update_now : Inport  Port=3
  update_next : Inport  Port=4
  Enable : EnablePort
  Subsystem : Subsystem
  Subsystem1 : Subsystem
  wires:
  tau_now_write/1 -> Subsystem/1(tau_now_write)
  tau_next_write/1 -> Subsystem1/1(tau_next_write)
  update_now/1 -> Subsystem/Enable
  update_next/1 -> Subsystem1/Enable

== system Hall_sensor_120deg_filter_org/hall_filter/software_ISR_routine/Subsystem ==
  Data Store Read : DataStoreRead  DataStoreName=tau_corr_next  IndexOptions=Index vector (dialog)  Indices=1  OutputSizes=1
  Data Store Write : DataStoreWrite  DataStoreName=tau_corr_now  IndexOptions=Index vector (dialog)  Indices=1  OutputSizes=1
  wires:
  Data Store Read/1 -> Data Store Write/1

== system Hall_sensor_120deg_filter_org/hall_filter/software_ISR_routine/Subsystem1 ==
  Constant : Constant  Value=-1
  Data Store Write1 : DataStoreWrite  DataStoreName=tau_corr_next  IndexOptions=Index vector (dialog)  Indices=1  OutputSizes=1
  wires:
  Constant/1 -> Data Store Write1/1

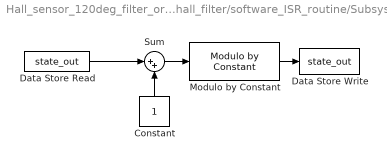
== system Hall_sensor_120deg_filter_org/hall_filter/software_ISR_routine/Subsystem2 ==
  Constant : Constant
  Data Store Read : DataStoreRead  DataStoreName=state_out  IndexOptions=Index vector (dialog)  Indices=1  OutputSizes=1
  Data Store Write : DataStoreWrite  DataStoreName=state_out  IndexOptions=Index vector (dialog)  Indices=1  OutputSizes=1
  Modulo by Constant : embmathops/Modulo by Constant  Denominator=6  SimulateUsing=Code generation
  Sum : Sum  Inputs=|++
  wires:
  Constant/1 -> Sum/2
  Data Store Read/1 -> Sum/1
  Sum/1 -> Modulo by Constant/1
  Modulo by Constant/1 -> Data Store Write/1

== system Hall_sensor_120deg_filter_org/hall_filter/software_ISR_routine/Subsystem3 ==
  Constant : Constant
  Data Store Read : DataStoreRead  DataStoreName=state_out  IndexOptions=Index vector (dialog)  Indices=1  OutputSizes=1
  Sum : Sum  Inputs=|++
  state_out : Outport
  wires:
  Data Store Read/1 -> Sum/1
  Sum/1 -> state_out/1
  Constant/1 -> Sum/2

== system Hall_sensor_120deg_filter_org/hall_filter/software_ISR_routine/Subsystem4 ==
  Constant : Constant  Value=0
  Data Store Write : DataStoreWrite  DataStoreName=first_time  IndexOptions=Index vector (dialog)  Indices=1  OutputSizes=1
  wires:
  Constant/1 -> Data Store Write/1

== system Hall_sensor_120deg_filter_org/hall_filter/hardware_ISR_routine/Atomic Subsystem/Subsystem ==
  tau_now_write : Inport
  update_now : EnablePort
  Data Store Write : DataStoreWrite  DataStoreName=tau_corr_now  IndexOptions=Index vector (dialog)  Indices=1  OutputSizes=1
  wires:
  tau_now_write/1 -> Data Store Write/1

== system Hall_sensor_120deg_filter_org/hall_filter/hardware_ISR_routine/Atomic Subsystem/Subsystem1 ==
  tau_next_write : Inport
  update_next : EnablePort
  Data Store Write1 : DataStoreWrite  DataStoreName=tau_corr_next  IndexOptions=Index vector (dialog)  Indices=1  OutputSizes=1
  wires:
  tau_next_write/1 -> Data Store Write1/1

== system Hall_sensor_120deg_filter_org/hall_filter/hardware_ISR_routine/Subsystem3/Subsystem ==
  tau_now_write : Inport
  update_now : EnablePort
  Data Store Write : DataStoreWrite  DataStoreName=tau_corr_now  IndexOptions=Index vector (dialog)  Indices=1  OutputSizes=1
  wires:
  tau_now_write/1 -> Data Store Write/1

== system Hall_sensor_120deg_filter_org/hall_filter/hardware_ISR_routine/Subsystem3/Subsystem1 ==
  tau_next_write : Inport
  update_next : EnablePort
  Data Store Write1 : DataStoreWrite  DataStoreName=tau_corr_next  IndexOptions=Index vector (dialog)  Indices=1  OutputSizes=1
  wires:
  tau_next_write/1 -> Data Store Write1/1

== matlab function Hall_sensor_120deg_filter_org/hall_filter/hardware_ISR_routine/MATLAB Function ==
  data: timer input; tau_now_out output; tau_vec input; tau_now input; tau_next input; tau_next_out output; update_now output; update_next output
function [tau_now_out, tau_next_out, update_now, update_next] = update_tau_vals_conditional_sim(timer, tau_vec, tau_now, tau_next)
[tau_now_out, tau_next_out, update_now, update_next] = update_tau_vals_conditional(timer, tau_vec, tau_now, tau_next);

== matlab function Hall_sensor_120deg_filter_org/hall sensors1 ==
  data: hall_errors input; theta_r input; H1 output; H2 output; H3 output
function [H1,H2,H3] = hall_sensor_sim(hall_errors, theta_r)
[H1,H2,H3] = hall_sensor(theta_r, hall_errors);
end

== matlab function Hall_sensor_120deg_filter_org/MATLAB Function2 ==
  data: H1 input; HALL_STATE output; H2 input; H3 input
function HALL_STATE = hall_to_statenum(H1,H2,H3)
HALL_STATE = 4*H1 + 2*H2 + H3;

== matlab function Hall_sensor_120deg_filter_org/qd-frame to stator ==
  data: fa output; fb output; fc output; fq input; fd input; theta input
function [fa,fb,fc] = K_mat_inv_sim(fq,fd,theta)
[fa,fb,fc] = K_mat_inv(fq,fd,theta);

== matlab function Hall_sensor_120deg_filter_org/stator to qd-frame ==
  data: fa input; fq output; fb input; fc input; theta input; fd output
function [fq,fd] = K_mat_sim(fa,fb,fc,theta)
[fq,fd] = K_mat(fa,fb,fc,theta);

== matlab function Hall_sensor_120deg_filter_org/back EMF ==
  data: fa output; fb output; fc output; fq input; fd input; theta input
function [fa,fb,fc] = K_mat_inv_sim_BEMF(fq,fd,theta)
[fa,fb,fc] = K_mat_inv(fq,fd,theta);

== matlab function Hall_sensor_120deg_filter_org/hall sensors ==
  data: hall_errors input; theta_r input; H1 output; H2 output; H3 output
function [H1,H2,H3] = hall_sensor_sim(hall_errors, theta_r)
[H1,H2,H3] = hall_sensor(theta_r, hall_errors);
end

== matlab function Hall_sensor_120deg_filter_org/controller_120 ==
  data: HALL_STATE input; T_vec output
function T_vec = controller_6step_120_sim(HALL_STATE)
T_vec = controller_6step_120(HALL_STATE);
end

== matlab function Hall_sensor_120deg_filter_org/MATLAB Function ==
  data: H1 input; HALL_STATE output; H2 input; H3 input
function HALL_STATE = hall_to_statenum(H1,H2,H3)
HALL_STATE = 4*H1 + 2*H2 + H3;

== matlab function Hall_sensor_120deg_filter_org/hall_filter/First trigger initialization/MATLAB Function ==
  data: num input; interval output
function interval = num_to_interval(num)
DICT = [5,3,4,1,6,2];
interval = DICT(num);

== matlab function Hall_sensor_120deg_filter_org/MATLAB Function1 ==
  data: omega_r input; f_Hz output
function f_Hz = avg_freq_sim(omega_r)
f_Hz = avg_freq(omega_r);

== matlab function Hall_sensor_120deg_filter_org/hall_filter/MATLAB Function ==
  data: H1 input; HALL_STATE output; H2 input; H3 input
function HALL_STATE = hall_to_statenum(H1,H2,H3)
HALL_STATE = 4*H1 + 2*H2 + H3;

== matlab function Hall_sensor_120deg_filter_org/hall_filter/MATLAB Function1 ==
  data: interval input; num output
function num = interval_to_num(interval)
DICT = [4,6,2,3,1,5];
if interval == 0
    num = 0;
else
    num = DICT(interval);
end
